simulink model "gm_ImageProcessingNoShift"  (R2023a)
settings: Solver=FixedStepDiscrete  StartTime=0.0  StopTime=2  RelTol=1e-3
undefined symbols (not defined in the file or in its folder): gray
libraries: hdlsllib x10, visionhdlio x6, visionsources x4, simulink x4
Description:
  | Sobel Edge Detection Using the MATLAB(R) Function Block
  | This example shows how to use HDL Coder(TM) to check,
  | generate, and verify HDL code for a Sobel Edge Detection
  | block built using the MATLAB Function block.
settings Model: Creator=The MathWorks, Inc.  LastModifiedBy=jms7664
settings SolverCC: AlgebraicLoopSolver=TrustRegion
settings DataIOCC: LimitDataPoints=on  SaveFormat=Array  SignalLogging=off  ReturnWorkspaceOutputs=off
settings OptimizationCC: BlockReduction=off  ConditionallyExecuteInputs=off  DefaultParameterBehavior=Inlined  ExpressionDepthLimit=2147483647  InitFltsAndDblsToZero=on  EfficientMapNaN2IntZero=off  LifeSpan=inf
settings DebuggingCC: AlgebraicLoopMsg=error  SaveWithParameterizedLinksMsg=none  UnderspecifiedInitializationDetection=Classic  MergeDetectMultiDrivingBlocksExec=none  SignalResolutionControl=TryResolveAllWithWarning  InheritedTsInSrcMsg=none  MultiTaskDSMMsg=warning  MultiTaskCondExecSysMsg=none  SingleTaskRateTransMsg=error  IntegerOverflowMsg=none  ParameterPrecisionLossMsg=none  FcnCallInpInsideContextMsg=warning  UnconnectedInputMsg=warning  UnconnectedOutputMsg=warning  UnconnectedLineMsg=warning  AllowSymbolicDim=off  StateNameClashWarn=warning  StrictBusMsg=ErrorOnBusTreatedAsVector  SFUnexpectedBacktrackingDiag=warning  SFNoUnconditionalDefaultTransitionDiag=warning  SFExecutionAtInitializationDiag=none  IntegerSaturationMsg=none  ArithmeticOperatorsInVariantConditions=warning
settings HardwareCC: ProdBitPerPointer=32  ProdBitPerSizeT=32  ProdBitPerPtrDiffT=32  ProdLargestAtomicFloat=None  ProdIntDivRoundTo=Undefined  ProdEndianess=Unspecified  ProdWordSize=32  ProdHWDeviceType=ASIC/FPGA  TargetHWDeviceType=32-bit Generic  ProdEqTarget=off
settings ModelReferenceCC: EnableRefExpFcnMdlSchedulingChecks=on  PropagateSignalLabelsOutOfModel=off
settings SFSimCC: SimUseLocalCustomCode=off  CustomCodeUndefinedFunction=UseInterfaceOnly
settings RTWCC: RTWUseLocalCustomCode=off  DLArmComputeVersion=19.05
settings CodeAppCC: StateflowObjectComments=on
settings GRTTargetCC: TargetFcnLib=ansi_tfl_tmw.mat  TargetLangStandard=C89/C90 (ANSI)  CombineOutputUpdateFcns=off  GRTInterface=on
settings ConfigComp: CovMetricSettings=dw  CovSaveCumulativeToWorkspaceVar=on  CovSaveSingleToWorkspaceVar=on  CovExternalEMLEnable=off

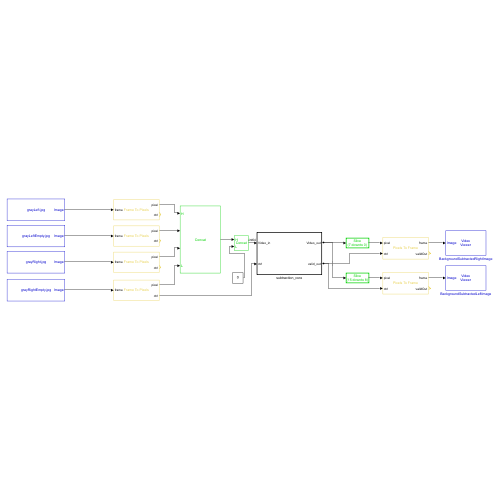
[thumbnail: Simulink's stored preview of the top-level diagram]
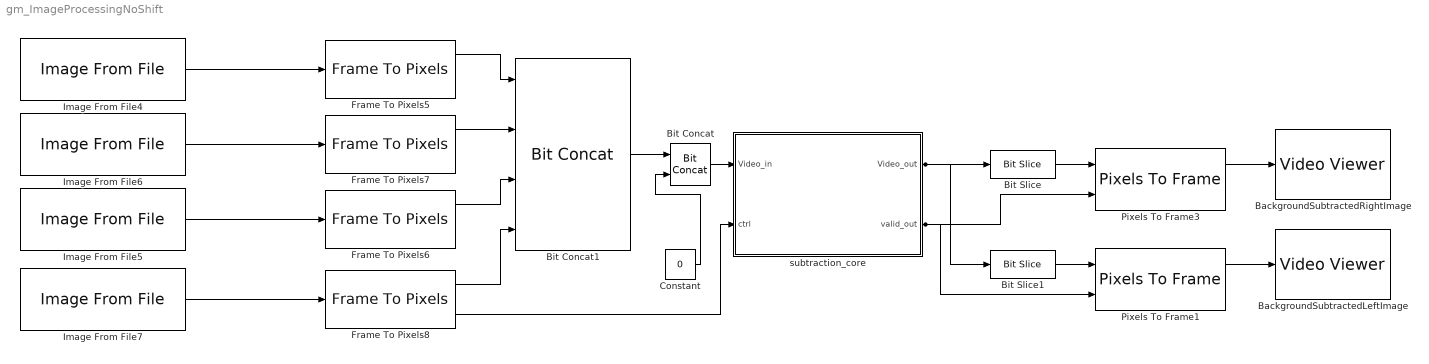
== system gm_ImageProcessingNoShift ==
  BackgroundSubtractedLeftImage : VideoViewer  colormapValue=gray(256)  FigPos=[0 1004 1920 930]
  BackgroundSubtractedRightImage : VideoViewer  colormapValue=gray(256)  FigPos=[0 1004 1920 930]
  Bit Concat : hdlsllib/Logic and Bit Operations/Bit Concat  numInputs=2
  Bit Concat1 : hdlsllib/Logic and Bit Operations/Bit Concat  numInputs=4
  Bit Slice : hdlsllib/Logic and Bit Operations/Bit Slice  lidx=7  ridx=0
  Bit Slice1 : hdlsllib/Logic and Bit Operations/Bit Slice  lidx=15  ridx=8
  Constant : Constant  Value=0  OutDataTypeStr=uint32  SampleTime=-1
  Frame To Pixels{5..8} (4 alike) : visionhdlio/Frame To Pixels  NumComponents=1  NumPixels=1  VideoFormat=Custom  ActivePixelsPerLine=752  ActiveVideoLines=480  TotalPixelsPerLine=752  TotalVideoLines=480  StartingActiveLine=1  FrontPorch=0  SampleTime=0  VideoFormatCache=Custom  ActivePixelsPerLineCache=752  ActiveVideoLinesCache=480  TotalPixelsPerLineCache=752  TotalVideoLinesCache=480  StartingActiveLineCache=1  FrontPorchCache=0
  Image From File4 : visionsources/Image From File  Tag=vipblks_nd  FileName=grayLeft.jpg  Ts=1  imagePorts=One multidimensional signal  OutPortLabels=R|G|B  ImageDataType=Inherit from input image  sdImageDataType=uint(8)  Signed=on  WordLength=16  FractionLengthMode=User-defined  FractionLength=15
  Image From File5 : visionsources/Image From File  Tag=vipblks_nd  FileName=grayRight.jpg  Ts=1  imagePorts=One multidimensional signal  OutPortLabels=R|G|B  ImageDataType=Inherit from input image  sdImageDataType=uint(8)  Signed=on  WordLength=16  FractionLengthMode=User-defined  FractionLength=15
  Image From File6 : visionsources/Image From File  Tag=vipblks_nd  FileName=grayLeftEmpty.jpg  Ts=1  imagePorts=One multidimensional signal  OutPortLabels=R|G|B  ImageDataType=Inherit from input image  sdImageDataType=uint(8)  Signed=on  WordLength=16  FractionLengthMode=User-defined  FractionLength=15
  Image From File7 : visionsources/Image From File  Tag=vipblks_nd  FileName=grayRightEmpty.jpg  Ts=1  imagePorts=One multidimensional signal  OutPortLabels=R|G|B  ImageDataType=Inherit from input image  sdImageDataType=uint(8)  Signed=on  WordLength=16  FractionLengthMode=User-defined  FractionLength=15
  Pixels To Frame1 : visionhdlio/Pixels To Frame  NumComponents=1  NumPixels=1  VideoFormat=Custom  ActivePixelsPerLine=R  ActiveVideoLines=C  TotalPixelsPerLine=R  TotalVideoLines=C  VideoFormatCache=Custom  ActivePixelsPerLineCache=R  ActiveVideoLinesCache=C  TotalPixelsPerLineCache=R  TotalVideoLinesCache=C
  Pixels To Frame3 : visionhdlio/Pixels To Frame  NumComponents=1  NumPixels=1  VideoFormat=Custom  ActivePixelsPerLine=R  ActiveVideoLines=C  TotalPixelsPerLine=R  TotalVideoLines=C  VideoFormatCache=Custom  ActivePixelsPerLineCache=R  ActiveVideoLinesCache=C  TotalPixelsPerLineCache=R  TotalVideoLinesCache=C
  subtraction_core : Subsystem  TreatAsAtomicUnit=on
  wires:
  Pixels To Frame1/1 -> BackgroundSubtractedLeftImage/1
  Pixels To Frame3/1 -> BackgroundSubtractedRightImage/1
  Bit Slice1/1 -> Pixels To Frame1/1
  Bit Slice/1 -> Pixels To Frame3/1
  subtraction_core/1(Video_out) -> Bit Slice1/1, Bit Slice/1
  subtraction_core/2(valid_out) -> Pixels To Frame1/2, Pixels To Frame3/2
  Bit Concat/1 -> subtraction_core/1(Video_in)
  Bit Concat1/1 -> Bit Concat/1
  Frame To Pixels8/2 -> subtraction_core/2(ctrl)
  Frame To Pixels8/1 -> Bit Concat1/4
  Frame To Pixels6/1 -> Bit Concat1/3
  Image From File7/1 -> Frame To Pixels8/1
  Image From File5/1 -> Frame To Pixels6/1
  Image From File6/1 -> Frame To Pixels7/1
  Image From File4/1 -> Frame To Pixels5/1
  Frame To Pixels5/1 -> Bit Concat1/1
  Frame To Pixels7/1 -> Bit Concat1/2
  Constant/1 -> Bit Concat/2

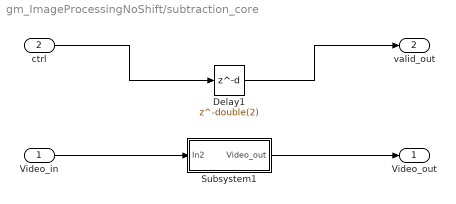
== system gm_ImageProcessingNoShift/subtraction_core ==
  Video_in : Inport  OutDataTypeStr=fixdt(0, 64, 0)  PortDimensions=1  SampleTime=2.77039007092199e-06
  ctrl : Inport  Port=2
  Delay1 : Delay  DelayLength=double(2)  SampleTime=2.77039007092199e-06
  Subsystem1 : Subsystem
  Video_out : Outport  SampleTime=2.77039007092199e-06  VectorParamsAs1DForOutWhenUnconnected=off
  valid_out : Outport  Port=2  VectorParamsAs1DForOutWhenUnconnected=off
  wires:
  Video_in/1 -> Subsystem1/1(In2)
  ctrl/1 -> Delay1/1
  Delay1/1 -> valid_out/1
  Subsystem1/1(Video_out) -> Video_out/1

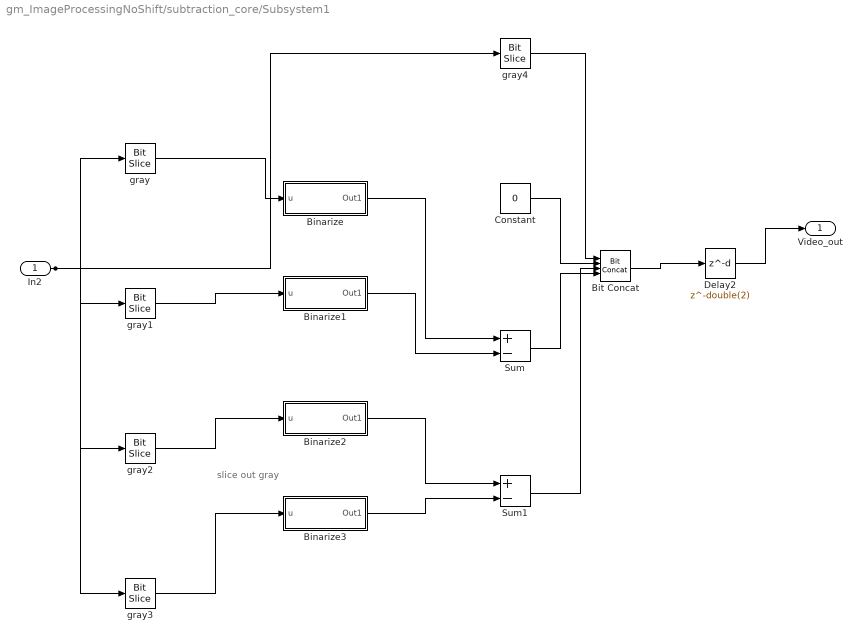
== system gm_ImageProcessingNoShift/subtraction_core/Subsystem1 ==
  note: slice out gray
  In2 : Inport  OutDataTypeStr=fixdt(0, 64, 0)  PortDimensions=1  SampleTime=2.77039007092199e-06
  Binarize : Subsystem
  Binarize1 : Subsystem
  Binarize2 : Subsystem
  Binarize3 : Subsystem
  Bit Concat : hdlsllib/Logic and Bit Operations/Bit Concat  numInputs=4
  Constant : Constant  Value=0  OutDataTypeStr=uint16  SampleTime=2.77039007092199e-06
  Delay2 : Delay  DelayLength=double(2)  InitialCondition=0  SampleTime=2.77039007092199e-06
  Sum : Sum  Inputs=+-  AccumDataTypeStr=fixdt(1, 9, 0)  OutDataTypeStr=uint8  SaturateOnIntegerOverflow=on  SampleTime=2.77039007092199e-06
  Sum1 : Sum  Inputs=+-  AccumDataTypeStr=fixdt(1, 9, 0)  OutDataTypeStr=uint8  SaturateOnIntegerOverflow=on  SampleTime=2.77039007092199e-06
  gray : hdlsllib/Logic and Bit Operations/Bit Slice  lidx=double(63)  ridx=double(56)
  gray1 : hdlsllib/Logic and Bit Operations/Bit Slice  lidx=double(55)  ridx=double(48)
  gray2 : hdlsllib/Logic and Bit Operations/Bit Slice  lidx=double(47)  ridx=double(40)
  gray3 : hdlsllib/Logic and Bit Operations/Bit Slice  lidx=double(39)  ridx=double(32)
  gray4 : hdlsllib/Logic and Bit Operations/Bit Slice  lidx=double(63)  ridx=double(32)
  Video_out : Outport  SampleTime=2.77039007092199e-06  InitialOutput=[0]
  wires:
  In2/1 -> gray4/1, gray3/1, gray2/1, gray1/1, gray/1
  Binarize/1(Out1) -> Sum/1
  Binarize1/1(Out1) -> Sum/2
  Binarize2/1(Out1) -> Sum1/1
  Binarize3/1(Out1) -> Sum1/2
  Bit Concat/1 -> Delay2/1
  Constant/1 -> Bit Concat/2
  Delay2/1 -> Video_out/1
  Sum/1 -> Bit Concat/4
  Sum1/1 -> Bit Concat/3
  gray/1 -> Binarize/1(u)
  gray1/1 -> Binarize1/1(u)
  gray2/1 -> Binarize2/1(u)
  gray3/1 -> Binarize3/1(u)
  gray4/1 -> Bit Concat/1

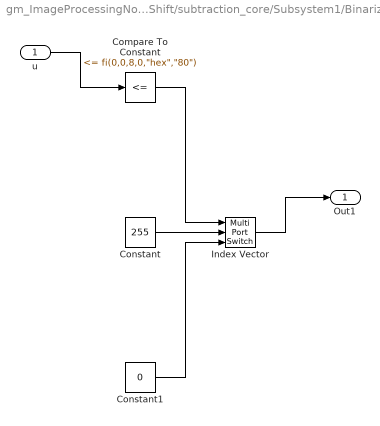
== system gm_ImageProcessingNoShift/subtraction_core/Subsystem1/Binarize ==
  u : Inport  OutDataTypeStr=uint8  PortDimensions=1  SampleTime=2.77039007092199e-06
  Compare To Constant : simulink/Logic and Bit Operations/Compare To Constant  relop=<=  const="fi(0,0,8,0,\"hex\",\"80\")"  OutDataTypeStr=boolean
  Constant : Constant  Value=255  OutDataTypeStr=uint8  SampleTime=2.77039007092199e-06
  Constant1 : Constant  Value=0  OutDataTypeStr=int8  SampleTime=2.77039007092199e-06
  Index Vector : MultiPortSwitch  DataPortOrder=Zero-based contiguous  Inputs=2  DiagnosticForDefault=None  zeroidx=on  OutDataTypeStr=uint8  SampleTime=2.77039007092199e-06  SaturateOnIntegerOverflow=off  InputSameDT=off
  Out1 : Outport  SampleTime=2.77039007092199e-06
  wires:
  u/1 -> Compare To Constant/1
  Compare To Constant/1 -> Index Vector/1
  Constant/1 -> Index Vector/2
  Constant1/1 -> Index Vector/3
  Index Vector/1 -> Out1/1

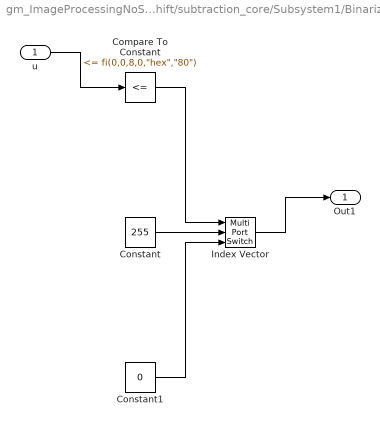
== system gm_ImageProcessingNoShift/subtraction_core/Subsystem1/Binarize1 ==
  u : Inport  OutDataTypeStr=uint8  PortDimensions=1  SampleTime=2.77039007092199e-06
  Compare To Constant : simulink/Logic and Bit Operations/Compare To Constant  relop=<=  const="fi(0,0,8,0,\"hex\",\"80\")"  OutDataTypeStr=boolean
  Constant : Constant  Value=255  OutDataTypeStr=uint8  SampleTime=2.77039007092199e-06
  Constant1 : Constant  Value=0  OutDataTypeStr=int8  SampleTime=2.77039007092199e-06
  Index Vector : MultiPortSwitch  DataPortOrder=Zero-based contiguous  Inputs=2  DiagnosticForDefault=None  zeroidx=on  OutDataTypeStr=uint8  SampleTime=2.77039007092199e-06  SaturateOnIntegerOverflow=off  InputSameDT=off
  Out1 : Outport  SampleTime=2.77039007092199e-06
  wires:
  u/1 -> Compare To Constant/1
  Compare To Constant/1 -> Index Vector/1
  Constant/1 -> Index Vector/2
  Constant1/1 -> Index Vector/3
  Index Vector/1 -> Out1/1

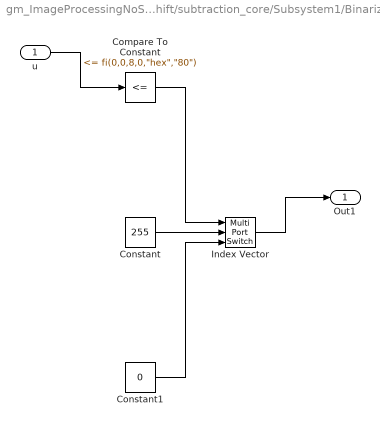
== system gm_ImageProcessingNoShift/subtraction_core/Subsystem1/Binarize2 ==
  u : Inport  OutDataTypeStr=uint8  PortDimensions=1  SampleTime=2.77039007092199e-06
  Compare To Constant : simulink/Logic and Bit Operations/Compare To Constant  relop=<=  const="fi(0,0,8,0,\"hex\",\"80\")"  OutDataTypeStr=boolean
  Constant : Constant  Value=255  OutDataTypeStr=uint8  SampleTime=2.77039007092199e-06
  Constant1 : Constant  Value=0  OutDataTypeStr=int8  SampleTime=2.77039007092199e-06
  Index Vector : MultiPortSwitch  DataPortOrder=Zero-based contiguous  Inputs=2  DiagnosticForDefault=None  zeroidx=on  OutDataTypeStr=uint8  SampleTime=2.77039007092199e-06  SaturateOnIntegerOverflow=off  InputSameDT=off
  Out1 : Outport  SampleTime=2.77039007092199e-06
  wires:
  u/1 -> Compare To Constant/1
  Compare To Constant/1 -> Index Vector/1
  Constant/1 -> Index Vector/2
  Constant1/1 -> Index Vector/3
  Index Vector/1 -> Out1/1

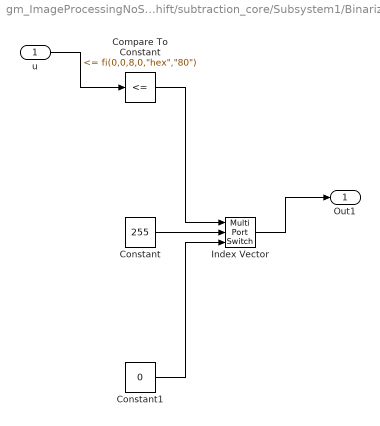
== system gm_ImageProcessingNoShift/subtraction_core/Subsystem1/Binarize3 ==
  u : Inport  OutDataTypeStr=uint8  PortDimensions=1  SampleTime=2.77039007092199e-06
  Compare To Constant : simulink/Logic and Bit Operations/Compare To Constant  relop=<=  const="fi(0,0,8,0,\"hex\",\"80\")"  OutDataTypeStr=boolean
  Constant : Constant  Value=255  OutDataTypeStr=uint8  SampleTime=2.77039007092199e-06
  Constant1 : Constant  Value=0  OutDataTypeStr=int8  SampleTime=2.77039007092199e-06
  Index Vector : MultiPortSwitch  DataPortOrder=Zero-based contiguous  Inputs=2  DiagnosticForDefault=None  zeroidx=on  OutDataTypeStr=uint8  SampleTime=2.77039007092199e-06  SaturateOnIntegerOverflow=off  InputSameDT=off
  Out1 : Outport  SampleTime=2.77039007092199e-06
  wires:
  u/1 -> Compare To Constant/1
  Compare To Constant/1 -> Index Vector/1
  Constant/1 -> Index Vector/2
  Constant1/1 -> Index Vector/3
  Index Vector/1 -> Out1/1
